simulink model "pmsm_sysid_debug"  (R2021a)
settings: Solver=VariableStepAuto  StartTime=0.0  StopTime=30  RelTol=1e-3
model workspace (MATLAB code in the model file):
  | np=4; % pole pairs
  | phiv=0.1167; % rotor flux, wb
  | Kt=3/2*np*phiv;
  | f=7.43e-5; %Nm/(rad/s), friction
  | J=1.74e-4; %kgm*m, inertia
  | L=0.004; %H, inductance
  | Ld=L;
  | Lq=L;
  | Rs=1.74; %Ohm, armature resistance
  | Kp=50; % Prop gain in inner PI
  | Ki=2500; % I gain in inner PI
  | Ti = Kp/Ki;
  | h = 1e-2; % Sampling period
  | wN = pi/h; % Nyquist freq
  | wBf = 0.7*wN; % Cutoff freq for AA filter
  | w0f = wBf/2.11; % AA filter param
undefined symbols (not defined in the file or in its folder): den, num
libraries: simulink x2
settings Model: Creator=kjartan  LastModifiedBy=kjartan
settings SolverCC: AlgebraicLoopSolver=TrustRegion
settings DataIOCC: ReturnWorkspaceOutputs=off
settings DebuggingCC: SFMachineParentedDataDiag=warning  ArithmeticOperatorsInVariantConditions=warning
settings SFSimCC: CustomCodeUndefinedFunction=UseInterfaceOnly

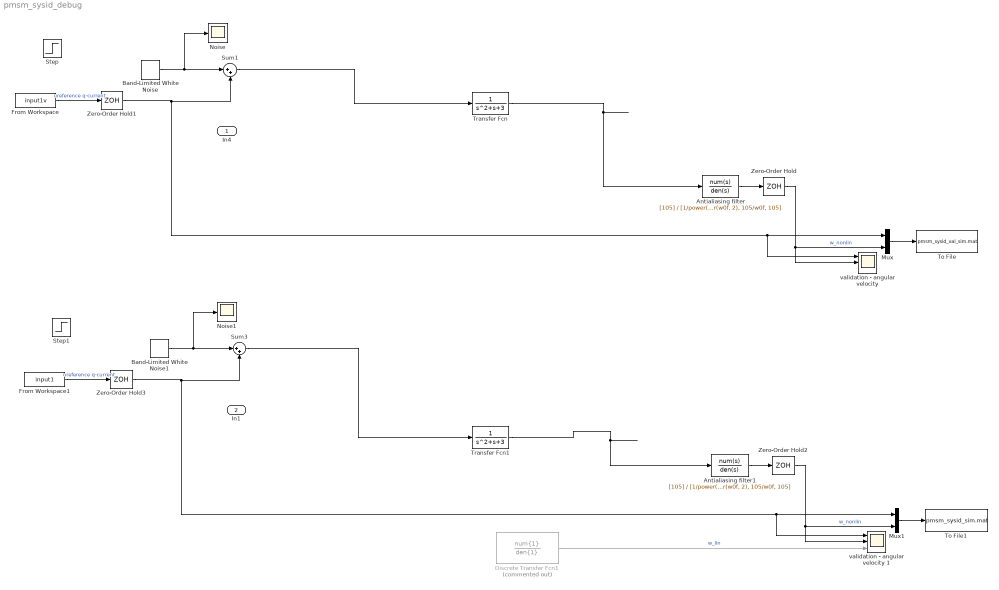
== system pmsm_sysid_debug ==
  In4 : Inport
  In1 : Inport  Port=2
  Antialiasing filter : TransferFcn  Numerator=[105]  Denominator=[1/power(w0f,4), 10/power(w0f, 3), 45/power(w0f, 2), 105/w0f, 105]
  Antialiasing filter1 : TransferFcn  Numerator=[105]  Denominator=[1/power(w0f,4), 10/power(w0f, 3), 45/power(w0f, 2), 105/w0f, 105]
  Band-Limited White Noise : simulink/Sources/Band-Limited White Noise  Cov=2  Ts=0.1  seed=[233412]
  Band-Limited White Noise1 : simulink/Sources/Band-Limited White Noise  Cov=2  Ts=0.1  seed=[233]
  Discrete Transfer Fcn1 : DiscreteTransferFcn  Commented=on  Numerator=num{1}  Denominator=den{1}  SampleTime=h
  From Workspace : FromWorkspace  VariableName=input1v  SampleTime=h
  From Workspace1 : FromWorkspace  VariableName=input1  SampleTime=h
  Mux : Mux  Inputs=2
  Mux1 : Mux  Inputs=2
  Noise : Scope
  Noise1 : Scope
  Step : Step  After=6  SampleTime=0
  Step1 : Step  After=6  SampleTime=0
  Sum1 : Sum  Inputs=|++
  Sum3 : Sum  Inputs=|++
  To File : ToFile  Filename=pmsm_sysid_val_sim.mat  MatrixName=uy  SaveFormat=Timeseries  SampleTime=h
  To File1 : ToFile  Filename=pmsm_sysid_sim.mat  MatrixName=uy  SaveFormat=Timeseries  SampleTime=h
  Transfer Fcn : TransferFcn  Denominator=[1 1 3]
  Transfer Fcn1 : TransferFcn  Denominator=[1 1 3]
  Zero-Order Hold{,1..3} (4 alike) : ZeroOrderHold  SampleTime=h
  "validation - angular velocity " : Scope  NumInputPorts=3
  validation - angular velocity 1 : Scope  NumInputPorts=3
  wires:
  Zero-Order Hold1/1 -> Sum1/2, "validation - angular velocity "/1, Mux/1
  Antialiasing filter/1 -> Zero-Order Hold/1
  Zero-Order Hold/1 -> Mux/2, "validation - angular velocity "/2  "w_nonlin"
  ? -> "validation - angular velocity "/3  "w_lin"
  Mux/1 -> To File/1
  From Workspace/1 -> Zero-Order Hold1/1  "ureference q-current"
  Band-Limited White Noise/1 -> Noise/1, Sum1/1
  From Workspace1/1 -> Zero-Order Hold3/1  "ureference q-current"
  Band-Limited White Noise1/1 -> Noise1/1, Sum3/1
  Zero-Order Hold3/1 -> Sum3/2, validation - angular velocity 1/1, Mux1/1
  Zero-Order Hold2/1 -> Mux1/2, validation - angular velocity 1/2  "w_nonlin"
  Antialiasing filter1/1 -> Zero-Order Hold2/1
  Discrete Transfer Fcn1/1 -> validation - angular velocity 1/3  "w_lin"
  Mux1/1 -> To File1/1
  Sum1/1 -> Transfer Fcn/1
  Sum3/1 -> Transfer Fcn1/1
  Transfer Fcn/1 -> Antialiasing filter/1
  Transfer Fcn1/1 -> Antialiasing filter1/1
